simulink model "QRD_RLS_model_top"  (R2020b)
settings: Solver=VariableStepAuto  StartTime=0.0  StopTime=10.0  RelTol=1e-3
libraries: dspsrcs4 x3, simulink x1
settings Model: Creator=jgentile  LastModifiedBy=johngentile

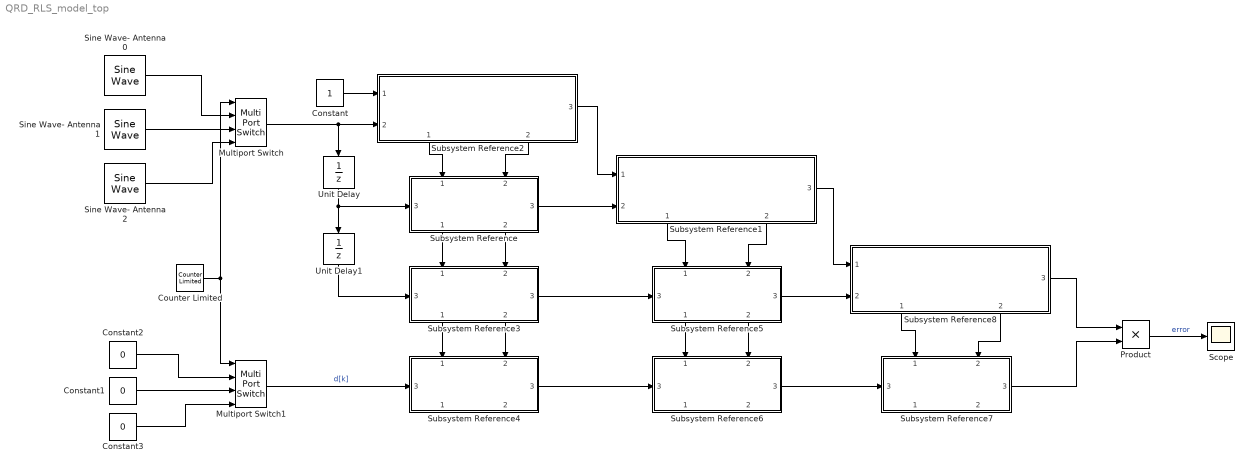
== system QRD_RLS_model_top ==
  Constant : Constant
  Constant1 : Constant  Value=0
  Constant2 : Constant  Value=0
  Constant3 : Constant  Value=0
  Counter Limited : simulink/Sources/Counter Limited  uplimit=2  tsamp=-1
  Multiport Switch : MultiPortSwitch
  Multiport Switch1 : MultiPortSwitch
  Product : Product
  Scope : Scope
  Sine Wave- Antenna 0 : dspsrcs4/Sine Wave  Amplitude=1  Frequency=100  Phase=0  SampleMode=Discrete  OutComplex=Complex  CompMethod=Trigonometric fcn  TableSize=Speed  SampleTime=1/1000  SamplesPerFrame=1  ResetState=Restart at time zero  OutputFrames=off  dataType=double  wordLen=16  udDataType=sfix(16)  fracBitsMode=Best precision  numFracBits=15  OutDataTypeStr=double  LastOutDataTypeStr=double
  Sine Wave- Antenna 1 : dspsrcs4/Sine Wave  Amplitude=1  Frequency=100  Phase=0  SampleMode=Discrete  OutComplex=Complex  CompMethod=Trigonometric fcn  TableSize=Speed  SampleTime=1/1000  SamplesPerFrame=1  ResetState=Restart at time zero  OutputFrames=off  dataType=double  wordLen=16  udDataType=sfix(16)  fracBitsMode=Best precision  numFracBits=15  OutDataTypeStr=double  LastOutDataTypeStr=double
  Sine Wave- Antenna 2 : dspsrcs4/Sine Wave  Amplitude=1  Frequency=100  Phase=0  SampleMode=Discrete  OutComplex=Complex  CompMethod=Trigonometric fcn  TableSize=Speed  SampleTime=1/1000  SamplesPerFrame=1  ResetState=Restart at time zero  OutputFrames=off  dataType=double  wordLen=16  udDataType=sfix(16)  fracBitsMode=Best precision  numFracBits=15  OutDataTypeStr=double  LastOutDataTypeStr=double
  Subsystem Reference{,3..7} (6 alike) : Subsystem  ReferencedSubsystem=internal_cell_givens
      settings: PortSchema="{\"entries\":[{\"content\":{\"sides\":[{\"content\":{\"connectorIds\":[\"In3\"]},\"type\":\"ConnectorPlacement.EquallySpacedRectSide\",\"uuid\":\"0239e4e7-44b6-4143-a587-38d4cded4ca6\"},{\"content\":{\"connectorIds\":[\"Out3\"],\"side\":\"RIGHT\"},\"type\":\"ConnectorPlacement.EquallySpacedRectSide\",\"uuid\":\"ea23c866-1a25-41e9-a0f2-3862af1c86e1\"},{\"content\":{\"connectorIds\":[\"In1\",\"In2\"],\"side\":\"TOP\"},\"type\":\"ConnectorPlacement.EquallySpacedRectSide\",\"uuid\":\"8a8bb13e-2e16-40e7-9ca3-19d820578314\"},{\"content\":{\"connectorIds\":[\"Out1\",\"Out2\"],\"side\":\"BOTTOM\"},\"type\":\"ConnectorPlacement.EquallySpacedRectSide\",\"uuid\":\"1be66ea9-adc8-4a43-a798-b14d6fcab7cd\"},{\"content\":{\"connectorIds\":[],\"side\":\"HIDDEN\"},\"type\":\"ConnectorPlacement.EquallySpacedRectSide\",\"uuid\":\"0fecdaf4-55de-420b-b554-931c979049af\"}]},\"type\":\"ConnectorPlacement.EquallySpacedConnector\",\"uuid\":\"70182f79-db57-400d-a53f-39946a20555a\"}],\"packageUris\":[\"http://schema.mathworks.com/mf0/Connector/R2020b\"],\"version\":\"1.0\"}"
  Subsystem Reference1 : Subsystem  ReferencedSubsystem=boundary_cell_givens
      settings: PortSchema="{\"entries\":[{\"content\":{\"sides\":[{\"content\":{\"connectorIds\":[\"In1\",\"In2\"]},\"type\":\"ConnectorPlacement.EquallySpacedRectSide\",\"uuid\":\"11c023aa-376d-416d-bfcd-8d7843f2be22\"},{\"content\":{\"connectorIds\":[\"Out3\"],\"side\":\"RIGHT\"},\"type\":\"ConnectorPlacement.EquallySpacedRectSide\",\"uuid\":\"1a04016b-daba-4444-ad99-d7273a1feb5b\"},{\"content\":{\"connectorIds\":[],\"side\":\"TOP\"},\"type\":\"ConnectorPlacement.EquallySpacedRectSide\",\"uuid\":\"dd6dcf65-02b5-4ffa-b5ff-7e58c587941b\"},{\"content\":{\"connectorIds\":[\"Out1\",\"Out2\"],\"side\":\"BOTTOM\"},\"type\":\"ConnectorPlacement.EquallySpacedRectSide\",\"uuid\":\"26ecda3d-5bd8-4d7b-b858-e25b16c314b4\"},{\"content\":{\"connectorIds\":[],\"side\":\"HIDDEN\"},\"type\":\"ConnectorPlacement.EquallySpacedRectSide\",\"uuid\":\"bd7630cc-a9b8-4021-b6b5-0e32bd520d7d\"}]},\"type\":\"ConnectorPlacement.EquallySpacedConnector\",\"uuid\":\"7bb81265-b299-46b6-8c47-6bc2be69935c\"}],\"packageUris\":[\"http://schema.mathworks.com/mf0/Connector/R2020b\"],\"version\":\"1.0\"}"
  Subsystem Reference2 : Subsystem  ReferencedSubsystem=boundary_cell_givens
      settings: PortSchema="{\"entries\":[{\"content\":{\"sides\":[{\"content\":{\"connectorIds\":[\"In1\",\"In2\"]},\"type\":\"ConnectorPlacement.EquallySpacedRectSide\",\"uuid\":\"11c023aa-376d-416d-bfcd-8d7843f2be22\"},{\"content\":{\"connectorIds\":[\"Out3\"],\"side\":\"RIGHT\"},\"type\":\"ConnectorPlacement.EquallySpacedRectSide\",\"uuid\":\"1a04016b-daba-4444-ad99-d7273a1feb5b\"},{\"content\":{\"connectorIds\":[],\"side\":\"TOP\"},\"type\":\"ConnectorPlacement.EquallySpacedRectSide\",\"uuid\":\"dd6dcf65-02b5-4ffa-b5ff-7e58c587941b\"},{\"content\":{\"connectorIds\":[\"Out1\",\"Out2\"],\"side\":\"BOTTOM\"},\"type\":\"ConnectorPlacement.EquallySpacedRectSide\",\"uuid\":\"26ecda3d-5bd8-4d7b-b858-e25b16c314b4\"},{\"content\":{\"connectorIds\":[],\"side\":\"HIDDEN\"},\"type\":\"ConnectorPlacement.EquallySpacedRectSide\",\"uuid\":\"bd7630cc-a9b8-4021-b6b5-0e32bd520d7d\"}]},\"type\":\"ConnectorPlacement.EquallySpacedConnector\",\"uuid\":\"7bb81265-b299-46b6-8c47-6bc2be69935c\"}],\"packageUris\":[\"http://schema.mathworks.com/mf0/Connector/R2020b\"],\"version\":\"1.0\"}"
  Subsystem Reference8 : Subsystem  ReferencedSubsystem=boundary_cell_givens
      settings: PortSchema="{\"entries\":[{\"content\":{\"sides\":[{\"content\":{\"connectorIds\":[\"In1\",\"In2\"]},\"type\":\"ConnectorPlacement.EquallySpacedRectSide\",\"uuid\":\"11c023aa-376d-416d-bfcd-8d7843f2be22\"},{\"content\":{\"connectorIds\":[\"Out3\"],\"side\":\"RIGHT\"},\"type\":\"ConnectorPlacement.EquallySpacedRectSide\",\"uuid\":\"1a04016b-daba-4444-ad99-d7273a1feb5b\"},{\"content\":{\"connectorIds\":[],\"side\":\"TOP\"},\"type\":\"ConnectorPlacement.EquallySpacedRectSide\",\"uuid\":\"dd6dcf65-02b5-4ffa-b5ff-7e58c587941b\"},{\"content\":{\"connectorIds\":[\"Out1\",\"Out2\"],\"side\":\"BOTTOM\"},\"type\":\"ConnectorPlacement.EquallySpacedRectSide\",\"uuid\":\"26ecda3d-5bd8-4d7b-b858-e25b16c314b4\"},{\"content\":{\"connectorIds\":[],\"side\":\"HIDDEN\"},\"type\":\"ConnectorPlacement.EquallySpacedRectSide\",\"uuid\":\"bd7630cc-a9b8-4021-b6b5-0e32bd520d7d\"}]},\"type\":\"ConnectorPlacement.EquallySpacedConnector\",\"uuid\":\"7bb81265-b299-46b6-8c47-6bc2be69935c\"}],\"packageUris\":[\"http://schema.mathworks.com/mf0/Connector/R2020b\"],\"version\":\"1.0\"}"
  Unit Delay : UnitDelay  SampleTime=-1  HasFrameUpgradeWarning=on
  Unit Delay1 : UnitDelay  SampleTime=-1  HasFrameUpgradeWarning=on
  wires:
  Subsystem Reference2/1 -> Subsystem Reference/1
  Subsystem Reference2/2 -> Subsystem Reference/2
  Subsystem Reference2/3 -> Subsystem Reference1/1
  Subsystem Reference/3 -> Subsystem Reference1/2
  Subsystem Reference/1 -> Subsystem Reference3/1
  Subsystem Reference/2 -> Subsystem Reference3/2
  Subsystem Reference3/1 -> Subsystem Reference4/1
  Subsystem Reference3/2 -> Subsystem Reference4/2
  Subsystem Reference3/3 -> Subsystem Reference5/3
  Subsystem Reference4/3 -> Subsystem Reference6/3
  Subsystem Reference1/1 -> Subsystem Reference5/1
  Subsystem Reference1/2 -> Subsystem Reference5/2
  Subsystem Reference5/1 -> Subsystem Reference6/1
  Subsystem Reference5/2 -> Subsystem Reference6/2
  Subsystem Reference1/3 -> Subsystem Reference8/1
  Subsystem Reference5/3 -> Subsystem Reference8/2
  Subsystem Reference6/3 -> Subsystem Reference7/3
  Subsystem Reference8/1 -> Subsystem Reference7/1
  Subsystem Reference8/2 -> Subsystem Reference7/2
  Subsystem Reference8/3 -> Product/1
  Subsystem Reference7/3 -> Product/2
  Product/1 -> Scope/1  "error"
  Constant/1 -> Subsystem Reference2/1
  Multiport Switch/1 -> Unit Delay/1, Subsystem Reference2/2
  Unit Delay/1 -> Unit Delay1/1, Subsystem Reference/3
  Unit Delay1/1 -> Subsystem Reference3/3
  Multiport Switch1/1 -> Subsystem Reference4/3  "d[k]"
  Sine Wave- Antenna 0/1 -> Multiport Switch/2
  Sine Wave- Antenna 1/1 -> Multiport Switch/3
  Sine Wave- Antenna 2/1 -> Multiport Switch/4
  Counter Limited/1 -> Multiport Switch1/1, Multiport Switch/1
  Constant1/1 -> Multiport Switch1/3
  Constant2/1 -> Multiport Switch1/2
  Constant3/1 -> Multiport Switch1/4
